simulink model "nn_xox"  (R2018b)
settings: Solver=VariableStepAuto  StartTime=0.0  StopTime=10.0  RelTol=1e-3
libraries: neural x4
settings Model: Creator=Mihail  LastModifiedBy=Mihail

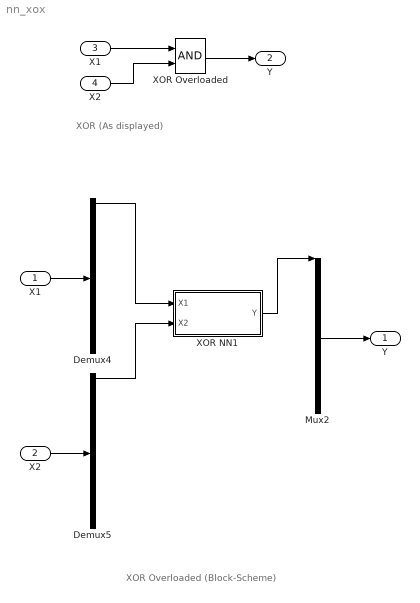
== system nn_xox ==
  note: XOR Overloaded
      | (Block-Scheme)
  note: XOR (As displayed)
  "X1   " : Inport
  "X2  " : Inport  Port=2
  X1 : Inport  Port=3
  X2 : Inport  Port=4
  Demux4 : Demux  Outputs=32
  Demux5 : Demux  Outputs=32
  Mux2 : Mux  Inputs=32
  XOR NN1 : Subsystem
  XOR Overloaded : Logic  AllPortsSameDT=off  OutDataTypeStr=boolean
  "Y  " : Outport
  Y : Outport  Port=2
  wires:
  XOR NN1/1(Y) -> Mux2/1
  Mux2/1 -> "Y  "/1
  "X2  "/1 -> Demux5/1
  Demux5/2 -> XOR NN1/2(X2)
  Demux4/2 -> XOR NN1/1(X1)
  "X1   "/1 -> Demux4/1
  X2/1 -> XOR Overloaded/2
  XOR Overloaded/1 -> Y/1
  X1/1 -> XOR Overloaded/1

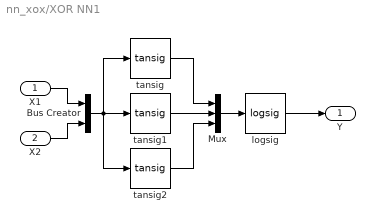
== system nn_xox/XOR NN1 ==
  X1 : Inport
  X2 : Inport  Port=2
  Bus Creator : BusCreator  Inputs=2
  Mux : Mux  Inputs=3
  logsig : neural/Transfer Functions/logsig
  tansig : neural/Transfer Functions/tansig
  tansig1 : neural/Transfer Functions/tansig
  tansig2 : neural/Transfer Functions/tansig
  Y : Outport
  wires:
  tansig2/1 -> Mux/3
  tansig1/1 -> Mux/2
  tansig/1 -> Mux/1
  Mux/1 -> logsig/1
  logsig/1 -> Y/1
  X1/1 -> Bus Creator/1
  X2/1 -> Bus Creator/2
  Bus Creator/1 -> tansig/1, tansig2/1, tansig1/1
